simulink model "test_route_planner"  (R2015b)
settings: Solver=FixedStepAuto  StartTime=0.0  StopTime=20  FixedStep=0.001  RelTol=1e-3
undefined symbols (not defined in the file or in its folder): sigbuilder_block
libraries: simulink x1
settings Model: Creator=rcasado  LastModifiedBy=rcasado

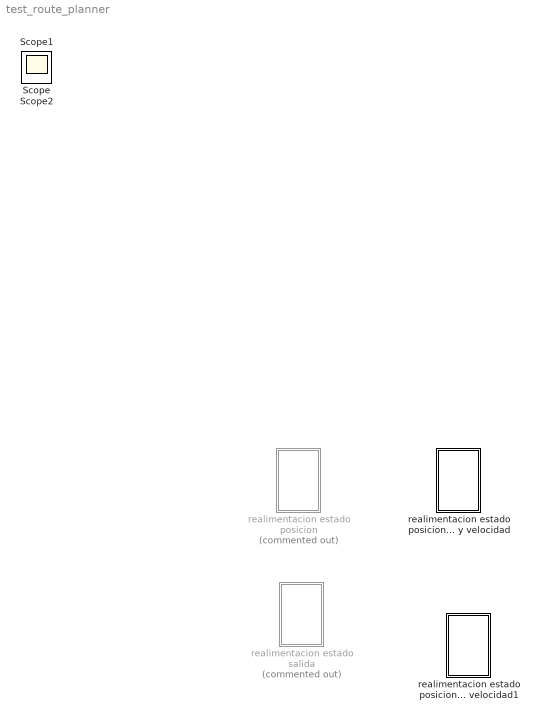
== system test_route_planner ==
  realimentacion estado posicion : Subsystem  Commented=on
  realimentacion estado posicion y velocidad : Subsystem
  realimentacion estado posicion y velocidad1 : Subsystem
  realimentacion estado salida : Subsystem  Commented=on
  Scope : Scope
  Scope1 : Scope
  Scope2 : Scope

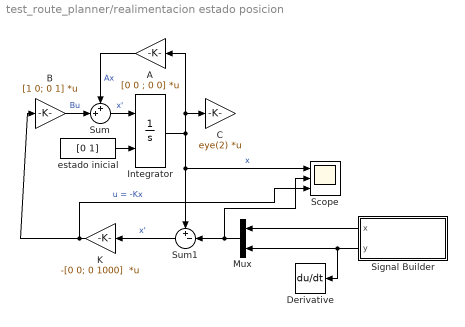
== system test_route_planner/realimentacion estado posicion ==
  A : Gain  Gain=[0 0 ; 0 0]  Multiplication=Matrix(K*u)
  B : Gain  Gain=[1 0; 0 1]  Multiplication=Matrix(K*u)
  C : Gain  Gain=eye(2)  Multiplication=Matrix(K*u)
  Derivative : Derivative
  Integrator : Integrator  InitialConditionSource=external  InitialCondition=[3; 1]
  K : Gain  Gain=-[0 0; 0 1000]  Multiplication=Matrix(K*u)
  Mux : Mux  Inputs=2
  Scope : Scope  NumInputPorts=3
  Signal Builder : Subsystem  Tag=STV Subsys  LoadFcn=sigbuilder_block('load');  StartFcn=sigbuilder_block('start');  StopFcn=sigbuilder_block('stop');  ClipboardFcn=sigbuilder_block('clipboard');  mask(Sigbuilder block){}
      mask help: Simulink:masks:SigbuilderBlock_MD
      mask init:
      | if ~strcmp(get_param(bdroot(gcbh),'SimulationStatus'),'stopped') tuvar = sigbuilder_block('maskInit'); end
      settings: CopyFcn=sigbuilder_block('copy');  DeleteFcn=sigbuilder_block('delete');  ModelCloseFcn=sigbuilder_block('modelClose');  PreSaveFcn=sigbuilder_block('preSave');  PauseFcn=sigbuilder_block('pause');  ContinueFcn=sigbuilder_block('continue');  NameChangeFcn=sigbuilder_block('namechange');  OpenFcn=sigbuilder_block('open',[564 136.2 550.8 400.2 ]);  CloseFcn=sigbuilder_block('close');
      mask Display: plot(0, 0, 100, 100,[2, 2, 32, 32, 2], [68, 8, 8, 68, 68],[32, 2], [38, 38], [32, 19, 2],[53, 60, 44], [32, 17, 17, 2],[16, 16, 31, 31]);txt = getActiveGroup(gcbh);text(2, 100, txt,'verticalAlignment', 'top');
  Sum : Sum  Inputs=++|
  Sum1 : Sum  Inputs=+-|
  estado inicial : Constant  Value=[0 1]
  wires:
  Integrator/1 -> A/1, C/1, Scope/1, Sum1/1  "x"
  Sum/1 -> Integrator/1  "x'"
  A/1 -> Sum/1  "Ax"
  B/1 -> Sum/2  "Bu"
  estado inicial/1 -> Integrator/2
  K/1 -> Scope/3, B/1  "u = -Kx"
  Mux/1 -> Scope/2, Sum1/2
  Sum1/1 -> K/1  "x'"
  Signal Builder/1(x) -> Mux/1
  Signal Builder/2(y) -> Derivative/1, Mux/2

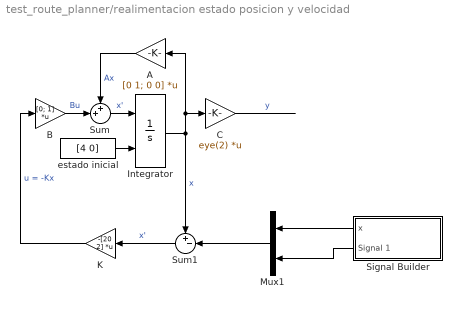
== system test_route_planner/realimentacion estado posicion y velocidad ==
  A : Gain  Gain=[0 1; 0 0]  Multiplication=Matrix(K*u)
  B : Gain  Gain=[0; 1]  Multiplication=Matrix(K*u)
  C : Gain  Gain=eye(2)  Multiplication=Matrix(K*u)
  Integrator : Integrator  InitialConditionSource=external  InitialCondition=[3; 1]
  K : Gain  Gain=-[20 2]  Multiplication=Matrix(K*u)
  Mux1 : Mux  Inputs=2
  Signal Builder : Subsystem  Tag=STV Subsys  LoadFcn=sigbuilder_block('load');  StartFcn=sigbuilder_block('start');  StopFcn=sigbuilder_block('stop');  ClipboardFcn=sigbuilder_block('clipboard');  mask(Sigbuilder block){}
      mask help: Simulink:masks:SigbuilderBlock_MD
      mask init:
      | if ~strcmp(get_param(bdroot(gcbh),'SimulationStatus'),'stopped') tuvar = sigbuilder_block('maskInit'); end
      settings: CopyFcn=sigbuilder_block('copy');  DeleteFcn=sigbuilder_block('delete');  ModelCloseFcn=sigbuilder_block('modelClose');  PreSaveFcn=sigbuilder_block('preSave');  PauseFcn=sigbuilder_block('pause');  ContinueFcn=sigbuilder_block('continue');  NameChangeFcn=sigbuilder_block('namechange');  OpenFcn=sigbuilder_block('open',[564 136.2 550.8 400.2 ]);  CloseFcn=sigbuilder_block('close');
      mask Display: plot(0, 0, 100, 100,[2, 2, 32, 32, 2], [68, 8, 8, 68, 68],[32, 2], [38, 38], [32, 19, 2],[53, 60, 44], [32, 17, 17, 2],[16, 16, 31, 31]);txt = getActiveGroup(gcbh);text(2, 100, txt,'verticalAlignment', 'top');
  Sum : Sum  Inputs=++|
  Sum1 : Sum  Inputs=+-|
  estado inicial : Constant  Value=[4 0]
  wires:
  Integrator/1 -> A/1, C/1, Sum1/1  "x"
  C/1 -> ?  "y"
  Sum/1 -> Integrator/1  "x'"
  A/1 -> Sum/1  "Ax"
  B/1 -> Sum/2  "Bu"
  estado inicial/1 -> Integrator/2
  K/1 -> B/1  "u = -Kx"
  Sum1/1 -> K/1  "x'"
  Signal Builder/1(x) -> Mux1/1
  Signal Builder/2(Signal 1) -> Mux1/2
  Mux1/1 -> Sum1/2

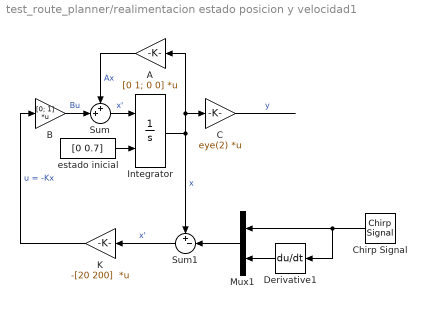
== system test_route_planner/realimentacion estado posicion y velocidad1 ==
  A : Gain  Gain=[0 1; 0 0]  Multiplication=Matrix(K*u)
  B : Gain  Gain=[0; 1]  Multiplication=Matrix(K*u)
  C : Gain  Gain=eye(2)  Multiplication=Matrix(K*u)
  Chirp Signal : simulink/Sources/Chirp Signal  f1=0.1  T=30  f2=0.5
  Derivative1 : Derivative
  Integrator : Integrator  InitialConditionSource=external  InitialCondition=[3; 1]
  K : Gain  Gain=-[20 200]  Multiplication=Matrix(K*u)
  Mux1 : Mux  Inputs=2
  Sum : Sum  Inputs=++|
  Sum1 : Sum  Inputs=+-|
  estado inicial : Constant  Value=[0 0.7]
  wires:
  Integrator/1 -> A/1, C/1, Sum1/1  "x"
  C/1 -> ?  "y"
  Sum/1 -> Integrator/1  "x'"
  A/1 -> Sum/1  "Ax"
  B/1 -> Sum/2  "Bu"
  estado inicial/1 -> Integrator/2
  K/1 -> B/1  "u = -Kx"
  Sum1/1 -> K/1  "x'"
  Chirp Signal/1 -> Derivative1/1, Mux1/1
  Derivative1/1 -> Mux1/2
  Mux1/1 -> Sum1/2

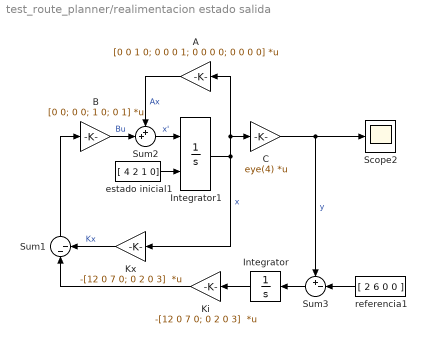
== system test_route_planner/realimentacion estado salida ==
  A : Gain  Gain=[0 0 1 0; 0 0 0 1; 0 0 0 0; 0 0 0 0]  Multiplication=Matrix(K*u)
  B : Gain  Gain=[0 0; 0 0; 1 0; 0 1]  Multiplication=Matrix(K*u)
  C : Gain  Gain=eye(4)  Multiplication=Matrix(K*u)
  Integrator : Integrator
  Integrator1 : Integrator  InitialConditionSource=external  InitialCondition=[3; 1]
  Ki : Gain  Gain=-[12 0 7 0; 0 2 0 3]  Multiplication=Matrix(K*u)
  Kx : Gain  Gain=-[12 0 7 0; 0 2 0 3]  Multiplication=Matrix(K*u)
  Scope2 : Scope
  Sum1 : Sum  Inputs=|--
  Sum2 : Sum  Inputs=++|
  Sum3 : Sum  Inputs=+-|
  estado inicial1 : Constant  Value=[ 4 2 1 0]
  referencia1 : Constant  Value=[ 2 6 0 0 ]
  wires:
  Integrator/1 -> Ki/1
  Sum3/1 -> Integrator/1
  Sum1/1 -> B/1
  C/1 -> Sum3/1, Scope2/1  "y"
  B/1 -> Sum2/2  "Bu"
  A/1 -> Sum2/1  "Ax"
  Kx/1 -> Sum1/2  "Kx"
  estado inicial1/1 -> Integrator1/2
  Sum2/1 -> Integrator1/1  "x'"
  referencia1/1 -> Sum3/2
  Integrator1/1 -> Kx/1, C/1, A/1  "x"
  Ki/1 -> Sum1/1

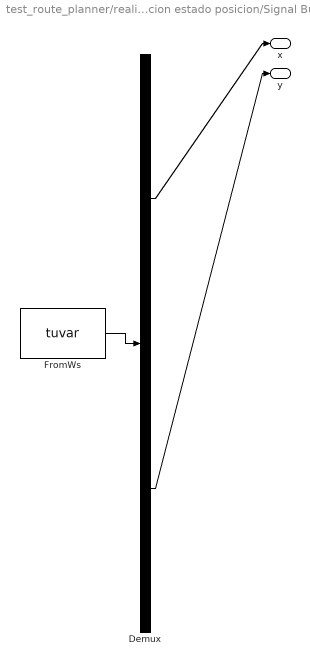
== system test_route_planner/realimentacion estado posicion/Signal Builder ==
  Demux : Demux  Tag=STV Demux  Outputs=2
  FromWs : FromWorkspace  Tag=STV FromWs  VariableName=tuvar  SampleTime=0
      SigBuilderData=|
      | common.afterFinalStr = 'Extrapolate'
      | common.sampleTime = 0
      | dataSet.timeRange = [0 20]
      | dataSet.name = 'Group 1'
      | sbobj.Groups.Name = 'Group 1'
      | sbobj.Groups.Signals(1).Name = 'x'
      | sbobj.Groups.Signals(1).XData = [0 20]
      | sbobj.Groups.Signals(1).YData = [0 0]
      | sbobj.Groups.Signals(2).Name = 'y'
      | sbobj.Groups.Signals(2).XData = [0 0.0808080808081 0.161616161616 0.242424242424 0.323232323232 0.40404040404 0.484848484848 0.565656565657 0.646464646465 0.727272727273 0.808080808081 0.888888888889 ... (249 elements, 1x249)]
      | sbobj.Groups.Signals(2).YData = [1 1.06342391966 1.12659245357 1.18925124436 1.25114798718 1.3120334457 1.37166245566 1.42979491209 1.4861967361 1.54064081746 1.59290792905 1.64278760969 ... (249 elements, 1x249)]
      | sbobj.Groups.TimeRange = [0 20]
  x : Outport  Tag=STV Outport
  y : Outport  Tag=STV Outport  Port=2
  wires:
  FromWs/1 -> Demux/1
  Demux/1 -> x/1
  Demux/2 -> y/1

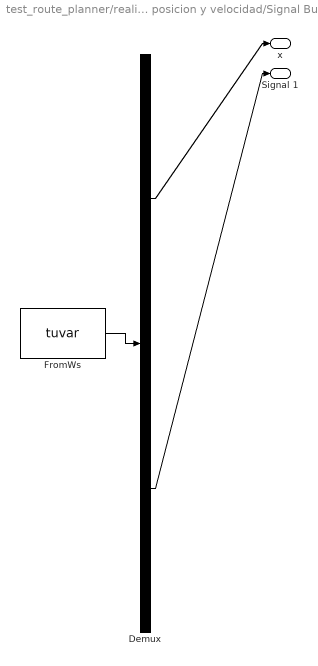
== system test_route_planner/realimentacion estado posicion y velocidad/Signal Builder ==
  Demux : Demux  Tag=STV Demux  Outputs=2
  FromWs : FromWorkspace  Tag=STV FromWs  VariableName=tuvar  SampleTime=0
      SigBuilderData=|
      | common.afterFinalStr = 'Extrapolate'
      | common.sampleTime = 0
      | dataSet.timeRange = [0 20]
      | dataSet.name = 'Group 1'
      | sbobj.Groups.Name = 'Group 1'
      | sbobj.Groups.Signals(1).Name = 'x'
      | sbobj.Groups.Signals(1).XData = [0 20]
      | sbobj.Groups.Signals(1).YData = [0 20]
      | sbobj.Groups.Signals(2).Name = 'Signal 1'
      | sbobj.Groups.Signals(2).XData = [0 20]
      | sbobj.Groups.Signals(2).YData = [1 1]
      | sbobj.Groups.TimeRange = [0 20]
  x : Outport  Tag=STV Outport
  Signal 1 : Outport  Tag=STV Outport  Port=2
  wires:
  FromWs/1 -> Demux/1
  Demux/1 -> x/1
  Demux/2 -> Signal 1/1
